simulink model "Rebuild"  (R2024b)
settings: Solver=VariableStepAuto  StartTime=0.0  StopTime=12  RelTol=1e-3
values from neighbouring files (symbols this model uses):
  A = 1.1    [RT14e_Parameters.m]    (also in RT15e_Parameters.m = 1.088; RT15evo_Parameters.m = 1.088)
  Aero_balance = 55    [RT14e_Parameters.m]    (also in RT15e_Parameters.m; RT15evo_Parameters.m)
  Aeromaps_ON = 0    [SIM_setup.m]
  air_density = 1.2    [SIM_setup.m]
  Balance_FW = Data_FW_STD(1:end,2)    [RT15e_Parameters.m]    (also in RT15evo_Parameters.m)
  Balance_R_11 = Data_R_11(1:end,2)    [RT15e_Parameters.m]    (also in RT15evo_Parameters.m)
  Br_coef_of_friction_F = 0.33    [RT14e_Parameters.m]    (also in RT15e_Parameters.m; RT15evo_Parameters.m)
  Br_coef_of_friction_R = 0.33    [RT14e_Parameters.m]    (also in RT15e_Parameters.m; RT15evo_Parameters.m)
  Br_pistons_area_F = 3617.26/1e6    (= 0.00361726)    [RT14e_Parameters.m]    (also in RT15e_Parameters.m; RT15evo_Parameters.m)
  Br_pistons_area_R = 2026.83/1e6    (= 0.00202683)    [RT14e_Parameters.m]    (also in RT15e_Parameters.m; RT15evo_Parameters.m)
  CdA = 1.31*A    (= 1.441)    [RT14e_Parameters.m]    (also in RT15e_Parameters.m = 1.700544; RT15evo_Parameters.m = 1.700544)
  CdA_FW = Data_FW_STD(1:end,3)    [RT15e_Parameters.m]    (also in RT15evo_Parameters.m)
  CdA_R_11 = Data_R_11(1:end,3)    [RT15e_Parameters.m]    (also in RT15evo_Parameters.m)
  ClA = 3.3*A    (= 3.63)    [RT14e_Parameters.m]    (also in RT15e_Parameters.m = 4.36288; RT15evo_Parameters.m = 4.36288)
  ClA_FW = Data_FW_STD(1:end,4)    [RT15e_Parameters.m]    (also in RT15evo_Parameters.m)
  ClA_R_11 = Data_R_11(1:end,4)    [RT15e_Parameters.m]    (also in RT15evo_Parameters.m)
  CoG_z = 0.35    [RT14e_Parameters.m]    (also in RT15e_Parameters.m = 0.28495; RT15evo_Parameters.m = 0.28495)
  Default_Fz_FL = Default_Fz_F/2 + (Default_Fz_F*CoG_y/Track_Front)    [RT14e_Parameters.m]    (also in RT15e_Parameters.m; RT15evo_Parameters.m)
  Default_Fz_FR = Default_Fz_F/2 - (Default_Fz_F*CoG_y/Track_Front)    [RT14e_Parameters.m]    (also in RT15e_Parameters.m; RT15evo_Parameters.m)
  Default_Fz_RL = Default_Fz_R/2 + (Default_Fz_R*CoG_y/Track_Rear)    [RT14e_Parameters.m]    (also in RT15e_Parameters.m; RT15evo_Parameters.m)
  Default_Fz_RR = Default_Fz_R/2 - (Default_Fz_R*CoG_y/Track_Rear)    [RT14e_Parameters.m]    (also in RT15e_Parameters.m; RT15evo_Parameters.m)
  Effective_br_disk_r_F = 0.0905    [RT14e_Parameters.m]    (also in RT15e_Parameters.m; RT15evo_Parameters.m)
  Effective_br_disk_r_R = 0.0895    [RT14e_Parameters.m]    (also in RT15e_Parameters.m; RT15evo_Parameters.m)
  Front_brake_balance = 0.0    (= 0)    [RT14e_Parameters.m]    (also in RT15e_Parameters.m; RT15evo_Parameters.m)
  Front_brake_pump_area = 153.94    [RT14e_Parameters.m]    (also in RT15e_Parameters.m; RT15evo_Parameters.m)
  Front_desired_brake_p_balance = 0.6    [RT14e_Parameters.m]    (also in RT15e_Parameters.m; RT15evo_Parameters.m)
  FW_Setup = Data_FW_STD(1:end,1)    [RT15e_Parameters.m]    (also in RT15evo_Parameters.m)
  Fx = Data_Fx(2:end,3:end)    [RT14e_Parameters.m]    (also in RT15e_Parameters.m; RT15evo_Parameters.m)
  Fy = Data_Fy(2:end,3:end)    [RT14e_Parameters.m]    (also in RT15e_Parameters.m; RT15evo_Parameters.m)
  Fz = Data_Fy(2:end,2)    [RT14e_Parameters.m]    (also in RT15e_Parameters.m; RT15evo_Parameters.m)
  g = 9.81    [SIM_setup.m]
  Gear_ratio = 12.9    [RT14e_Parameters.m]    (also in RT15e_Parameters.m; RT15evo_Parameters.m)
  Iz_wehicle = 120    [RT14e_Parameters.m]    (also in RT15e_Parameters.m; RT15evo_Parameters.m)
  Iz_wheel = 0.15    [RT14e_Parameters.m]    (also in RT15e_Parameters.m; RT15evo_Parameters.m)
  Lf = Wheelbase - CoG_x    (= 0.77)    [RT14e_Parameters.m]    (also in RT15e_Parameters.m = 0.7504; RT15evo_Parameters.m = 0.7504)
  LLTD = 0.45    [RT14e_Parameters.m]    (also in RT15e_Parameters.m = 0.55; RT15evo_Parameters.m = 0.55)
  Lock_brake_balance = false    [RT14e_Parameters.m]    (also in RT15e_Parameters.m; RT15evo_Parameters.m)
  Lr = Wheelbase - Lf    (= 0.755)    [RT14e_Parameters.m]    (also in RT15e_Parameters.m = 0.7746; RT15evo_Parameters.m = 0.7746)
  Mass = Vehicle_mass + Driver_mass    (= 290)    [RT14e_Parameters.m]    (also in RT15e_Parameters.m = 265; RT15evo_Parameters.m)
  Motor_maximum_power = 35366    [RT14e_Parameters.m]    (also in RT15e_Parameters.m; RT15evo_Parameters.m)
  RB_torque_setting_1 = -2    [RT14e_Parameters.m]    (also in RT15e_Parameters.m; RT15evo_Parameters.m)
  RB_torque_setting_10 = -20    [RT14e_Parameters.m]    (also in RT15e_Parameters.m; RT15evo_Parameters.m)
  RB_torque_setting_2 = -4    [RT14e_Parameters.m]    (also in RT15e_Parameters.m; RT15evo_Parameters.m)
  RB_torque_setting_3 = -6    [RT14e_Parameters.m]    (also in RT15e_Parameters.m; RT15evo_Parameters.m)
  RB_torque_setting_4 = -8    [RT14e_Parameters.m]    (also in RT15e_Parameters.m; RT15evo_Parameters.m)
  RB_torque_setting_5 = -10    [RT14e_Parameters.m]    (also in RT15e_Parameters.m; RT15evo_Parameters.m)
  RB_torque_setting_6 = -12    [RT14e_Parameters.m]    (also in RT15e_Parameters.m; RT15evo_Parameters.m)
  RB_torque_setting_7 = -14    [RT14e_Parameters.m]    (also in RT15e_Parameters.m; RT15evo_Parameters.m)
  RB_torque_setting_8 = -16    [RT14e_Parameters.m]    (also in RT15e_Parameters.m; RT15evo_Parameters.m)
  RB_torque_setting_9 = -18    [RT14e_Parameters.m]    (also in RT15e_Parameters.m; RT15evo_Parameters.m)
  Rear_brake_pump_area = 198.56    [RT14e_Parameters.m]    (also in RT15e_Parameters.m; RT15evo_Parameters.m)
  Roll_Angle_11 = Data_R_11(1:end,1)    [RT15e_Parameters.m]    (also in RT15evo_Parameters.m)
  SA = Data_Fy(1,3:end)    [RT14e_Parameters.m]    (also in RT15e_Parameters.m; RT15evo_Parameters.m)
  SR = Data_Fx(1,3:end)    [RT14e_Parameters.m]    (also in RT15e_Parameters.m; RT15evo_Parameters.m)
  start_acc_x = double(start_acc_x_ts.Data)    [SIM_setup.m]
  start_acc_y = double(start_acc_y_ts.Data)    [SIM_setup.m]
  start_time = 1188    [SIM_setup.m]
  start_velocity_x = double(start_velocity_x_ts.Data)    [SIM_setup.m]
  start_velocity_y = double(start_velocity_y_ts.Data)    [SIM_setup.m]
  start_yaw_acc = double(start_yaw_acc_ts.Data)    [SIM_setup.m]
  start_yaw_rate = double(start_yaw_rate_ts.Data)    [SIM_setup.m]
  Static_Camber_FL = 0    [RT14e_Parameters.m]    (also in RT15e_Parameters.m; RT15evo_Parameters.m)
  Static_Camber_FR = 0    [RT14e_Parameters.m]    (also in RT15e_Parameters.m; RT15evo_Parameters.m)
  Static_Camber_RL = 0    [RT14e_Parameters.m]    (also in RT15e_Parameters.m; RT15evo_Parameters.m)
  Static_Camber_RR = 0    [RT14e_Parameters.m]    (also in RT15e_Parameters.m; RT15evo_Parameters.m)
  Static_Toe_FL = 0    [RT14e_Parameters.m]    (also in RT15e_Parameters.m; RT15evo_Parameters.m)
  Static_Toe_FR = 0    [RT14e_Parameters.m]    (also in RT15e_Parameters.m; RT15evo_Parameters.m)
  Static_Toe_RL = 0    [RT14e_Parameters.m]    (also in RT15e_Parameters.m; RT15evo_Parameters.m)
  Static_Toe_RR = 0    [RT14e_Parameters.m]    (also in RT15e_Parameters.m; RT15evo_Parameters.m)
  Steering_Angle_FL = Data_Steering(1:end,2)    [RT14e_Parameters.m]    (also in RT15e_Parameters.m; RT15evo_Parameters.m)
  Steering_Angle_FR = Data_Steering(1:end,3)    [RT14e_Parameters.m]    (also in RT15e_Parameters.m; RT15evo_Parameters.m)
  Steering_Wheel_Angle = Data_Steering(1:end,1)    [RT14e_Parameters.m]    (also in RT15e_Parameters.m; RT15evo_Parameters.m)
  Tire_radius = 0.203    [RT14e_Parameters.m]    (also in RT15e_Parameters.m; RT15evo_Parameters.m)
  Torque_limit_2 = Motor_maximum_torque*0.2    (= 5.82)    [RT14e_Parameters.m]    (also in RT15e_Parameters.m; RT15evo_Parameters.m)
  Torque_limit_3 = Motor_maximum_torque*0.3    (= 8.73)    [RT14e_Parameters.m]    (also in RT15e_Parameters.m; RT15evo_Parameters.m)
  Torque_limit_4 = Motor_maximum_torque*0.4    (= 11.64)    [RT14e_Parameters.m]    (also in RT15e_Parameters.m; RT15evo_Parameters.m)
  Torque_limit_5 = Motor_maximum_torque*0.5    (= 14.55)    [RT14e_Parameters.m]    (also in RT15e_Parameters.m; RT15evo_Parameters.m)
  Torque_limit_6 = Motor_maximum_torque*0.6    (= 17.46)    [RT14e_Parameters.m]    (also in RT15e_Parameters.m; RT15evo_Parameters.m)
  Torque_limit_7 = Motor_maximum_torque*0.7    (= 20.37)    [RT14e_Parameters.m]    (also in RT15e_Parameters.m; RT15evo_Parameters.m)
  Torque_limit_8 = Motor_maximum_torque*0.8    (= 23.28)    [RT14e_Parameters.m]    (also in RT15e_Parameters.m; RT15evo_Parameters.m)
  Torque_limit_9 = 29.1    [RT14e_Parameters.m]    (also in RT15e_Parameters.m; RT15evo_Parameters.m)
  Torque_limit_max = Motor_maximum_torque    (= 29.1)    [RT14e_Parameters.m]    (also in RT15e_Parameters.m; RT15evo_Parameters.m)
  Torque_limit_min = Motor_maximum_torque*0.1    (= 2.91)    [RT14e_Parameters.m]    (also in RT15e_Parameters.m; RT15evo_Parameters.m)
  Torque_limit_set = 10    [RT14e_Parameters.m]    (also in RT15e_Parameters.m; RT15evo_Parameters.m)
  Track_Front = 1.2    [RT14e_Parameters.m]    (also in RT15e_Parameters.m; RT15evo_Parameters.m)
  Track_Rear = 1.18    [RT14e_Parameters.m]    (also in RT15e_Parameters.m; RT15evo_Parameters.m)
  TV_ON = 0    [SIM_setup.m]
  TV_RB_understeer_gradient_1 = -0.5    [RT14e_Parameters.m]    (also in RT15e_Parameters.m; RT15evo_Parameters.m)
  TV_RB_understeer_gradient_10 = 0.005    [RT14e_Parameters.m]    (also in RT15e_Parameters.m; RT15evo_Parameters.m)
  TV_RB_understeer_gradient_2 = -0.1    [RT14e_Parameters.m]    (also in RT15e_Parameters.m; RT15evo_Parameters.m)
  TV_RB_understeer_gradient_3 = 0.08    [RT14e_Parameters.m]    (also in RT15e_Parameters.m; RT15evo_Parameters.m)
  TV_RB_understeer_gradient_4 = 0.06    [RT14e_Parameters.m]    (also in RT15e_Parameters.m; RT15evo_Parameters.m)
  TV_RB_understeer_gradient_5 = 0.05    [RT14e_Parameters.m]    (also in RT15e_Parameters.m; RT15evo_Parameters.m)
  TV_RB_understeer_gradient_6 = 0.04    [RT14e_Parameters.m]    (also in RT15e_Parameters.m; RT15evo_Parameters.m)
  TV_RB_understeer_gradient_7 = 0.03    [RT14e_Parameters.m]    (also in RT15e_Parameters.m; RT15evo_Parameters.m)
  TV_RB_understeer_gradient_8 = 0.02    [RT14e_Parameters.m]    (also in RT15e_Parameters.m; RT15evo_Parameters.m)
  TV_RB_understeer_gradient_9 = 0.01    [RT14e_Parameters.m]    (also in RT15e_Parameters.m; RT15evo_Parameters.m)
  TV_understeer_gradient_1 = -0.5    [RT14e_Parameters.m]    (also in RT15e_Parameters.m; RT15evo_Parameters.m)
  TV_understeer_gradient_10 = 0.002    [RT14e_Parameters.m]    (also in RT15e_Parameters.m; RT15evo_Parameters.m)
  TV_understeer_gradient_2 = -0.1    [RT14e_Parameters.m]    (also in RT15e_Parameters.m; RT15evo_Parameters.m)
  TV_understeer_gradient_3 = 0.06    [RT14e_Parameters.m]    (also in RT15e_Parameters.m; RT15evo_Parameters.m)
  TV_understeer_gradient_4 = 0.05    [RT14e_Parameters.m]    (also in RT15e_Parameters.m; RT15evo_Parameters.m)
  TV_understeer_gradient_5 = 0.04    [RT14e_Parameters.m]    (also in RT15e_Parameters.m; RT15evo_Parameters.m)
  TV_understeer_gradient_6 = 0.03    [RT14e_Parameters.m]    (also in RT15e_Parameters.m; RT15evo_Parameters.m)
  TV_understeer_gradient_7 = 0.02    [RT14e_Parameters.m]    (also in RT15e_Parameters.m; RT15evo_Parameters.m)
  TV_understeer_gradient_8 = 0.01    [RT14e_Parameters.m]    (also in RT15e_Parameters.m; RT15evo_Parameters.m)
  TV_understeer_gradient_9 = 0.005    [RT14e_Parameters.m]    (also in RT15e_Parameters.m; RT15evo_Parameters.m)
  Vx_APPS_ON = 1    [SIM_setup.m]
  Wheel_rolling_resistance = 0.055    [RT14e_Parameters.m]    (also in RT15e_Parameters.m; RT15evo_Parameters.m)
  Wheelbase = 1.525    [RT14e_Parameters.m]    (also in RT15e_Parameters.m; RT15evo_Parameters.m)
undefined symbols (not defined in the file or in its folder): Actual_Torque_Value_RL, Actual_Torque_Value_RR, aero_balance, APPS, Brake_Pressure_Front, Brake_Pressure_Rear, Cl, lateral_load_transfer_distribution, maths_GPS_Velocity, Max_Torque, rad, s, Steering_position, tire_radius, wheel_base, Wheel_Speed_RL, Wheel_Speed_RR, Xsens_MTI_670_accX, Xsens_MTI_670_accY, Xsens_MTI_670_gyrZ
libraries: simulink x30, simulink_extras x11, slpidlib x9, dspstat3 x4, slrealtimeloglib x1, aerolibconvert2 x1
(part 5 of 6)

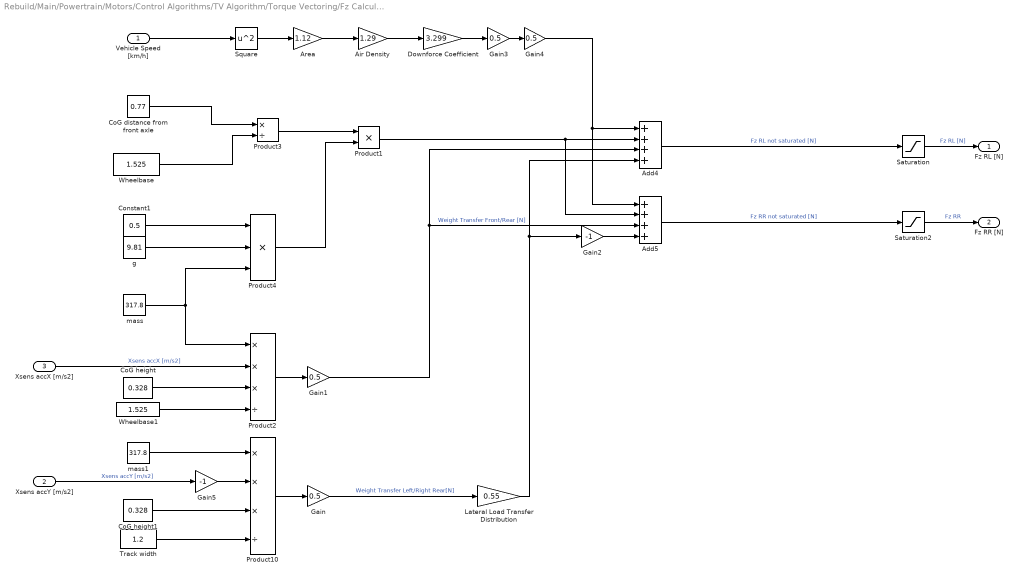
== system Rebuild/Main/Powertrain/Motors/Control Algorithms/TV Algorithm/Torque Vectoring/Fz Calculation ==
  Vehicle Speed [km/h] : Inport
  Xsens accY [m/s2] : Inport  Port=2
  Xsens accX [m/s2] : Inport  Port=3
  Add4 : Sum  Inputs=++++
  Add5 : Sum  Inputs=++++
  Air Density : Gain  Gain=1.29
  Area : Gain  Gain=1.12
  CoG distance from front axle : Constant  Value=0.77
  CoG height : Constant  Value=0.328
  CoG height1 : Constant  Value=0.328
  Constant1 : Constant  Value=0.5
  Downforce Coefficient : Gain  Gain=3.299
  Gain{,1,3..4} (4 alike) : Gain  Gain=0.5
  Gain2 : Gain  Gain=-1
  Gain5 : Gain  Gain=-1
  Lateral Load Transfer Distribution : Gain  Gain=0.55
  Product1 : Product
  Product10 : Product  Inputs=***/
  Product2 : Product  Inputs=***/
  Product3 : Product  Inputs=*/
  Product4 : Product  Inputs=3
  Saturation : Saturate  UpperLimit=10000  LowerLimit=0
  Saturation2 : Saturate  UpperLimit=10000  LowerLimit=0
  Square : Math  Operator=square
  Track width : Constant  Value=1.2
  Wheelbase : Constant  Value=1.525
  Wheelbase1 : Constant  Value=1.525
  g : Constant  Value=9.81
  mass : Constant  Value=317.8
  mass1 : Constant  Value=317.8
  Fz RL [N] : Outport
  Fz RR [N] : Outport  Port=2
  wires:
  Xsens accX [m/s2]/1 -> Product2/2  "Xsens accX [m/s2]"
  Xsens accY [m/s2]/1 -> Gain5/1  "Xsens accY [m/s2]"
  Add5/1 -> Saturation2/1  "Fz RR not saturated [N]"
  Saturation2/1 -> Fz RR [N]/1  "Fz RR"
  Saturation/1 -> Fz RL [N]/1  "Fz RL [N]"
  Add4/1 -> Saturation/1  "Fz RL not saturated [N]"
  Product2/1 -> Gain1/1
  Product3/1 -> Product1/1
  CoG distance from front axle/1 -> Product3/1
  Wheelbase1/1 -> Product2/4
  CoG height/1 -> Product2/3
  mass/1 -> Product4/3, Product2/1
  Product10/1 -> Gain/1
  Constant1/1 -> Product4/1
  Track width/1 -> Product10/4
  g/1 -> Product4/2
  Product4/1 -> Product1/2
  Wheelbase/1 -> Product3/2
  CoG height1/1 -> Product10/3
  mass1/1 -> Product10/1
  Gain/1 -> Lateral Load Transfer Distribution/1  "Weight Transfer Left/Right Rear[N]"
  Gain1/1 -> Add4/3, Add5/3  "Weight Transfer Front/Rear [N]"
  Lateral Load Transfer Distribution/1 -> Add4/4, Gain2/1
  Product1/1 -> Add4/2, Add5/2
  Gain2/1 -> Add5/4
  Vehicle Speed [km/h]/1 -> Square/1
  Square/1 -> Area/1
  Area/1 -> Air Density/1
  Air Density/1 -> Downforce Coefficient/1
  Gain3/1 -> Gain4/1
  Gain4/1 -> Add5/1, Add4/1
  Downforce Coefficient/1 -> Gain3/1
  Gain5/1 -> Product10/2

== system Rebuild/Main/Powertrain/Motors/Control Algorithms/TV Algorithm/Torque Vectoring/RB Torque Difference Calculation ==
  Desired Yaw Rate TV [deg/s] : Inport
  SWS VD Parameter 4 : Inport  Port=2
  " " : Constant  Value=1.2
  "  " : Constant  Value=13
  "   " : Constant  Value=tire_radius
  Abs : Abs  SaturateOnIntegerOverflow=off
  Compare To Constant : simulink/Logic and Bit Operations/Compare To Constant  relop===  const=1  OutDataTypeStr=boolean
  Compare To Constant1 : simulink/Logic and Bit Operations/Compare To Constant  relop===  const=2  OutDataTypeStr=boolean
  Divide3 : Product  Inputs=**
  Divide4 : Product  Inputs=*/
  Divide5 : Product  Inputs=**
  Gain : Gain  Gain=40
  Gain1 : Gain  Gain=0.5
  Gain2 : Gain  Gain=-1
  OR : Logic  Operator=OR  IconShape=distinctive  AllPortsSameDT=off  OutDataTypeStr=boolean
  Saturation : Saturate  UpperLimit=29.1  LowerLimit=0
  Switch : Switch  Criteria=u2 > Threshold  SaturateOnIntegerOverflow=off  InputSameDT=off
  Torque Difference RB [Nm] : Outport
  wires:
  Gain2/1 -> Switch/1
  Switch/1 -> Torque Difference RB [Nm]/1
  Saturation/1 -> Switch/3, Gain2/1  "Torque Difference [Nm]"
  SWS VD Parameter 4/1 -> Compare To Constant/1, Compare To Constant1/1
  Compare To Constant/1 -> OR/1
  Compare To Constant1/1 -> OR/2
  Abs/1 -> Saturation/1
  Gain1/1 -> Abs/1
  Divide4/1 -> Gain1/1
  "   "/1 -> Divide3/1
  " "/1 -> Divide5/2
  Divide5/1 -> Divide4/2
  "  "/1 -> Divide5/1
  Gain/1 -> Divide3/2
  Desired Yaw Rate TV [deg/s]/1 -> Gain/1
  Divide3/1 -> Divide4/1
  OR/1 -> Switch/2

== system Rebuild/Main/Powertrain/Motors/Control Algorithms/TV Algorithm/Torque Vectoring/RB Yaw Rate Calculation ==
  SWS VD Parameter 4 : Inport
  Wheel Angle F [deg] : Inport  Port=2
  Vehicle Speed [km/h] : Inport  Port=3
  " " : Constant  Value=wheel_base
  Add : Sum
  Divide : Product  Inputs=**/
  Divide1 : Product  Inputs=**
  File Log : slrealtimeloglib/File Log  decimation=1  inputProcessing=Elements as channels (sample based)
  Square : Math  Operator=square
  Understeer Gradeint Selection : Subsystem
  Desired Yaw Rate TV RB [deg/s] : Outport
  wires:
  SWS VD Parameter 4/1 -> Understeer Gradeint Selection/1(SWS VD Parameter 4)
  Wheel Angle F [deg]/1 -> Divide/1
  Add/1 -> Divide/3
  Divide1/1 -> Add/2
  Understeer Gradeint Selection/1(Understeer Gradient) -> Divide1/2
  Square/1 -> Divide1/1
  Vehicle Speed [km/h]/1 -> Divide/2, Square/1
  Divide/1 -> Desired Yaw Rate TV RB [deg/s]/1, File Log/1  "Desired Yaw Rate TV [deg/s]"
  " "/1 -> Add/1

== system Rebuild/Main/Powertrain/Motors/Control Algorithms/TV Algorithm/Torque Vectoring/Subsystem ==
  Torque After TV RL [Nm] not saturated : Inport
  SWS VD Parameter 6 : Inport  Port=2
  Torque After TV RR [Nm] not saturated : Inport  Port=3
  Bus Selector : BusSelector  OutputSignals=Torque After TV RL [Nm],Torque After TV RR [Nm]
  Merge : Merge  Inputs=11
  Switch Case : SwitchCase  CaseConditions={1,2,3,4,5,6,7,8,9,10}
  Switch Case Action Subsystem : Subsystem  TreatAsAtomicUnit=on
  Switch Case Action Subsystem1 : Subsystem  TreatAsAtomicUnit=on
  Switch Case Action Subsystem10 : Subsystem  TreatAsAtomicUnit=on
  Switch Case Action Subsystem2 : Subsystem  TreatAsAtomicUnit=on
  Switch Case Action Subsystem3 : Subsystem  TreatAsAtomicUnit=on
  Switch Case Action Subsystem4 : Subsystem  TreatAsAtomicUnit=on
  Switch Case Action Subsystem5 : Subsystem  TreatAsAtomicUnit=on
  Switch Case Action Subsystem6 : Subsystem  TreatAsAtomicUnit=on
  Switch Case Action Subsystem7 : Subsystem  TreatAsAtomicUnit=on
  Switch Case Action Subsystem8 : Subsystem  TreatAsAtomicUnit=on
  Switch Case Action Subsystem9 : Subsystem  TreatAsAtomicUnit=on
  Torque After TV RL [Nm] : Outport
  Torque After TV RR [Nm] : Outport  Port=2
  wires:
  Switch Case Action Subsystem/1(Out1) -> Merge/1
  Switch Case Action Subsystem1/1(Out1) -> Merge/2
  Switch Case Action Subsystem2/1(Out1) -> Merge/3
  Switch Case Action Subsystem3/1(Out1) -> Merge/4
  Switch Case Action Subsystem4/1(Out1) -> Merge/5
  Switch Case Action Subsystem5/1(Out1) -> Merge/6
  Switch Case Action Subsystem6/1(Out1) -> Merge/7
  Switch Case Action Subsystem7/1(Out1) -> Merge/8
  Switch Case Action Subsystem8/1(Out1) -> Merge/9
  Switch Case Action Subsystem9/1(Out1) -> Merge/10
  Switch Case Action Subsystem10/1(Out1) -> Merge/11
  SWS VD Parameter 6/1 -> Switch Case/1
  Switch Case/1 -> Switch Case Action Subsystem/Action
  Switch Case/2 -> Switch Case Action Subsystem1/Action
  Switch Case/3 -> Switch Case Action Subsystem2/Action
  Switch Case/4 -> Switch Case Action Subsystem3/Action
  Switch Case/5 -> Switch Case Action Subsystem4/Action
  Switch Case/6 -> Switch Case Action Subsystem5/Action
  Switch Case/7 -> Switch Case Action Subsystem6/Action
  Switch Case/8 -> Switch Case Action Subsystem7/Action
  Switch Case/9 -> Switch Case Action Subsystem8/Action
  Switch Case/10 -> Switch Case Action Subsystem9/Action
  Switch Case/11 -> Switch Case Action Subsystem10/Action
  Torque After TV RL [Nm] not saturated/1 -> Switch Case Action Subsystem10/1(Torque After TV RL [Nm] not saturated), Switch Case Action Subsystem9/1(Torque After TV RL [Nm] not saturated), Switch Case Action Subsystem8/1(Torque After TV RL [Nm] not saturated), Switch Case Action Subsystem7/1(Torque After TV RL [Nm] not saturated), Switch Case Action Subsystem6/1(Torque After TV RL [Nm] not saturated), Switch Case Action Subsystem5/1(Torque After TV RL [Nm] not saturated), Switch Case Action Subsystem3/1(Torque After TV RL [Nm] not saturated), Switch Case Action Subsystem1/1(Torque After TV RL [Nm] not saturated), Switch Case Action Subsystem/1(Torque After TV RL [Nm] not saturated), Switch Case Action Subsystem2/1(Torque After TV RL [Nm] not saturated), Switch Case Action Subsystem4/1(Torque After TV RL [Nm] not saturated)
  Torque After TV RR [Nm] not saturated/1 -> Switch Case Action Subsystem/2(Torque After TV RR [Nm] not saturated), Switch Case Action Subsystem1/2(Torque After TV RR [Nm] not saturated), Switch Case Action Subsystem2/2(Torque After TV RR [Nm] not saturated), Switch Case Action Subsystem3/2(Torque After TV RR [Nm] not saturated), Switch Case Action Subsystem4/2(Torque After TV RR [Nm] not saturated), Switch Case Action Subsystem5/2(Torque After TV RR [Nm] not saturated), Switch Case Action Subsystem6/2(Torque After TV RR [Nm] not saturated), Switch Case Action Subsystem7/2(Torque After TV RR [Nm] not saturated), Switch Case Action Subsystem8/2(Torque After TV RR [Nm] not saturated), Switch Case Action Subsystem9/2(Torque After TV RR [Nm] not saturated), Switch Case Action Subsystem10/2(Torque After TV RR [Nm] not saturated)
  Merge/1 -> Bus Selector/1
  Bus Selector/1 -> Torque After TV RL [Nm]/1  "<Torque After TV RL [Nm]>"
  Bus Selector/2 -> Torque After TV RR [Nm]/1  "<Torque After TV RR [Nm]>"

== system Rebuild/Main/Powertrain/Motors/Control Algorithms/TV Algorithm/Torque Vectoring/Subsystem1 ==
  Torque After TV RL [Nm] not saturated : Inport
  Torque After TV RR [Nm] not saturated : Inport  Port=2
  SWS VD Parameter 6 : Inport  Port=3
  Bus Selector : BusSelector  OutputSignals=Torque After TV RL [Nm],Torque After TV RR [Nm]
  Merge : Merge  Inputs=11
  Switch Case : SwitchCase  CaseConditions={1,2,3,4,5,6,7,8,9,10}
  Switch Case Action Subsystem : Subsystem  TreatAsAtomicUnit=on
  Switch Case Action Subsystem1 : Subsystem  TreatAsAtomicUnit=on
  Switch Case Action Subsystem10 : Subsystem  TreatAsAtomicUnit=on
  Switch Case Action Subsystem2 : Subsystem  TreatAsAtomicUnit=on
  Switch Case Action Subsystem3 : Subsystem  TreatAsAtomicUnit=on
  Switch Case Action Subsystem4 : Subsystem  TreatAsAtomicUnit=on
  Switch Case Action Subsystem5 : Subsystem  TreatAsAtomicUnit=on
  Switch Case Action Subsystem6 : Subsystem  TreatAsAtomicUnit=on
  Switch Case Action Subsystem7 : Subsystem  TreatAsAtomicUnit=on
  Switch Case Action Subsystem8 : Subsystem  TreatAsAtomicUnit=on
  Switch Case Action Subsystem9 : Subsystem  TreatAsAtomicUnit=on
  Torque After TV RL [Nm] : Outport
  Torque After TV RR [Nm] : Outport  Port=2
  wires:
  Bus Selector/2 -> Torque After TV RR [Nm]/1  "<Torque After TV RR [Nm]>"
  Bus Selector/1 -> Torque After TV RL [Nm]/1  "<Torque After TV RL [Nm]>"
  Merge/1 -> Bus Selector/1
  Torque After TV RR [Nm] not saturated/1 -> Switch Case Action Subsystem10/2(Torque After TV RR [Nm] not saturated), Switch Case Action Subsystem9/2(Torque After TV RR [Nm] not saturated), Switch Case Action Subsystem8/2(Torque After TV RR [Nm] not saturated), Switch Case Action Subsystem7/2(Torque After TV RR [Nm] not saturated), Switch Case Action Subsystem6/2(Torque After TV RR [Nm] not saturated), Switch Case Action Subsystem5/2(Torque After TV RR [Nm] not saturated), Switch Case Action Subsystem4/2(Torque After TV RR [Nm] not saturated), Switch Case Action Subsystem3/2(Torque After TV RR [Nm] not saturated), Switch Case Action Subsystem2/2(Torque After TV RR [Nm] not saturated), Switch Case Action Subsystem1/2(Torque After TV RR [Nm] not saturated), Switch Case Action Subsystem/2(Torque After TV RR [Nm] not saturated)
  Torque After TV RL [Nm] not saturated/1 -> Switch Case Action Subsystem4/1(Torque After TV RL [Nm] not saturated), Switch Case Action Subsystem2/1(Torque After TV RL [Nm] not saturated), Switch Case Action Subsystem/1(Torque After TV RL [Nm] not saturated), Switch Case Action Subsystem1/1(Torque After TV RL [Nm] not saturated), Switch Case Action Subsystem3/1(Torque After TV RL [Nm] not saturated), Switch Case Action Subsystem5/1(Torque After TV RL [Nm] not saturated), Switch Case Action Subsystem6/1(Torque After TV RL [Nm] not saturated), Switch Case Action Subsystem7/1(Torque After TV RL [Nm] not saturated), Switch Case Action Subsystem8/1(Torque After TV RL [Nm] not saturated), Switch Case Action Subsystem9/1(Torque After TV RL [Nm] not saturated), Switch Case Action Subsystem10/1(Torque After TV RL [Nm] not saturated)
  Switch Case/11 -> Switch Case Action Subsystem10/Action
  Switch Case/10 -> Switch Case Action Subsystem9/Action
  Switch Case/9 -> Switch Case Action Subsystem8/Action
  Switch Case/8 -> Switch Case Action Subsystem7/Action
  Switch Case/7 -> Switch Case Action Subsystem6/Action
  Switch Case/6 -> Switch Case Action Subsystem5/Action
  Switch Case/5 -> Switch Case Action Subsystem4/Action
  Switch Case/4 -> Switch Case Action Subsystem3/Action
  Switch Case/3 -> Switch Case Action Subsystem2/Action
  Switch Case/2 -> Switch Case Action Subsystem1/Action
  Switch Case/1 -> Switch Case Action Subsystem/Action
  SWS VD Parameter 6/1 -> Switch Case/1
  Switch Case Action Subsystem10/1(Out1) -> Merge/11
  Switch Case Action Subsystem9/1(Out1) -> Merge/10
  Switch Case Action Subsystem8/1(Out1) -> Merge/9
  Switch Case Action Subsystem7/1(Out1) -> Merge/8
  Switch Case Action Subsystem6/1(Out1) -> Merge/7
  Switch Case Action Subsystem5/1(Out1) -> Merge/6
  Switch Case Action Subsystem4/1(Out1) -> Merge/5
  Switch Case Action Subsystem3/1(Out1) -> Merge/4
  Switch Case Action Subsystem2/1(Out1) -> Merge/3
  Switch Case Action Subsystem1/1(Out1) -> Merge/2
  Switch Case Action Subsystem/1(Out1) -> Merge/1

== system Rebuild/Main/Powertrain/Motors/Control Algorithms/TV Algorithm/Torque Vectoring/Subsystem2 ==
  Brakes : Inport
  In3 : Inport  Port=2
  AND2 : Logic  IconShape=distinctive  AllPortsSameDT=off  OutDataTypeStr=boolean
  Bus Selector : BusSelector  OutputSignals=Front,Rear
  Compare To Constant3 : simulink/Logic and Bit Operations/Compare To Constant  relop=>=  const=5  OutDataTypeStr=boolean
  Compare To Constant4 : simulink/Logic and Bit Operations/Compare To Constant  relop=>=  const=5  OutDataTypeStr=boolean
  OR : Logic  Operator=OR  IconShape=distinctive  AllPortsSameDT=off  OutDataTypeStr=boolean
  Regen Braking Check : Outport
  wires:
  AND2/1 -> Regen Braking Check/1  "Regen Braking Check"
  Compare To Constant3/1 -> OR/2
  OR/1 -> AND2/1
  Compare To Constant4/1 -> OR/1
  In3/1 -> AND2/2
  Bus Selector/1 -> Compare To Constant4/1  "<Front>"
  Brakes/1 -> Bus Selector/1
  Bus Selector/2 -> Compare To Constant3/1  "<Rear>"

== system Rebuild/Main/Powertrain/Motors/Control Algorithms/TV Algorithm/Torque Vectoring/TV Activation ==
  Wheel Angle F [deg] : Inport
  Vehicle Speed [km/h] : Inport  Port=2
  SWS VD Setup 3 : Inport  Port=3
  Regen Braking Check : Inport  Port=4
  R2D Status : Inport  Port=5
  AND : Logic  Inputs=5  IconShape=distinctive  AllPortsSameDT=off  OutDataTypeStr=boolean
  Compare To Constant : simulink/Logic and Bit Operations/Compare To Constant  relop=>=  const=3  OutDataTypeStr=boolean
  Compare To Constant1 : simulink/Logic and Bit Operations/Compare To Constant  relop=<=  const=-3  OutDataTypeStr=boolean
  Compare To Constant2 : simulink/Logic and Bit Operations/Compare To Constant  relop=>  const=-1  OutDataTypeStr=boolean
  NOT : Logic  Operator=NOT  IconShape=distinctive  AllPortsSameDT=off  OutDataTypeStr=boolean
  OR1 : Logic  Operator=OR  IconShape=distinctive  AllPortsSameDT=off  OutDataTypeStr=boolean
  TV Active : Outport
  wires:
  AND/1 -> TV Active/1
  R2D Status/1 -> AND/2
  SWS VD Setup 3/1 -> AND/1
  Compare To Constant1/1 -> OR1/2
  Compare To Constant/1 -> OR1/1
  Wheel Angle F [deg]/1 -> Compare To Constant/1, Compare To Constant1/1
  Vehicle Speed [km/h]/1 -> Compare To Constant2/1
  Compare To Constant2/1 -> AND/3
  OR1/1 -> AND/4
  Regen Braking Check/1 -> NOT/1
  NOT/1 -> AND/5

== system Rebuild/Main/Powertrain/Motors/Control Algorithms/TV Algorithm/Torque Vectoring/TV RB Activation ==
  R2D Status : Inport
  Regen Braking Check : Inport  Port=2
  Vehicle Speed [km/h] : Inport  Port=3
  SWS VD Setup 4 : Inport  Port=4
  Wheel Angle F [deg] : Inport  Port=5
  AND : Logic  Inputs=5  IconShape=distinctive  AllPortsSameDT=off  OutDataTypeStr=boolean
  Compare To Constant : simulink/Logic and Bit Operations/Compare To Constant  relop=>=  const=3  OutDataTypeStr=boolean
  Compare To Constant1 : simulink/Logic and Bit Operations/Compare To Constant  relop=<=  const=-3  OutDataTypeStr=boolean
  Compare To Constant2 : simulink/Logic and Bit Operations/Compare To Constant  relop=>  const=10  OutDataTypeStr=boolean
  OR1 : Logic  Operator=OR  IconShape=distinctive  AllPortsSameDT=off  OutDataTypeStr=boolean
  TV RB Active : Outport
  wires:
  OR1/1 -> AND/4
  Wheel Angle F [deg]/1 -> Compare To Constant1/1, Compare To Constant/1
  Compare To Constant/1 -> OR1/1
  Compare To Constant1/1 -> OR1/2
  SWS VD Setup 4/1 -> AND/1
  R2D Status/1 -> AND/2
  AND/1 -> TV RB Active/1
  Vehicle Speed [km/h]/1 -> Compare To Constant2/1
  Compare To Constant2/1 -> AND/3
  Regen Braking Check/1 -> AND/5

== system Rebuild/Main/Powertrain/Motors/Control Algorithms/TV Algorithm/Torque Vectoring/Torque Difference Calculation ==
  Desired Yaw Rate TV [deg/s] : Inport
  SWS VD Setup 15 : Inport  Port=2
  SWS VD Parameter 3 : Inport  Port=3
  " " : Constant  Value=1.2
  "  " : Constant  Value=13
  "   " : Constant  Value=tire_radius
  AND : Logic  IconShape=distinctive  AllPortsSameDT=off  OutDataTypeStr=boolean
  Abs : Abs  SaturateOnIntegerOverflow=off
  Compare To Constant : simulink/Logic and Bit Operations/Compare To Constant  relop===  const=1  OutDataTypeStr=boolean
  Compare To Constant1 : simulink/Logic and Bit Operations/Compare To Constant  relop===  const=2  OutDataTypeStr=boolean
  Compare To Constant2 : simulink/Logic and Bit Operations/Compare To Constant  relop===  const=0  OutDataTypeStr=boolean
  Divide3 : Product  Inputs=**
  Divide4 : Product  Inputs=*/
  Divide5 : Product  Inputs=**
  Gain : Gain  Gain=40
  Gain1 : Gain  Gain=0.5
  Gain2 : Gain  Gain=-1
  OR : Logic  Operator=OR  IconShape=distinctive  AllPortsSameDT=off  OutDataTypeStr=boolean
  Saturation : Saturate  UpperLimit=Torque_limit_max  LowerLimit=0
  Switch : Switch  Criteria=u2 > Threshold  SaturateOnIntegerOverflow=off  InputSameDT=off
  Torque Difference [Nm] : Outport
  wires:
  Divide3/1 -> Divide4/1
  Desired Yaw Rate TV [deg/s]/1 -> Gain/1
  Gain/1 -> Divide3/2
  "  "/1 -> Divide5/1
  Divide5/1 -> Divide4/2
  " "/1 -> Divide5/2
  "   "/1 -> Divide3/1
  Divide4/1 -> Gain1/1
  Gain1/1 -> Abs/1
  Abs/1 -> Saturation/1
  Compare To Constant1/1 -> OR/2
  Compare To Constant/1 -> OR/1
  SWS VD Parameter 3/1 -> Compare To Constant1/1, Compare To Constant/1
  Saturation/1 -> Gain2/1, Switch/3  "Torque Difference [Nm]"
  Switch/1 -> Torque Difference [Nm]/1
  Gain2/1 -> Switch/1
  OR/1 -> AND/1
  SWS VD Setup 15/1 -> Compare To Constant2/1
  AND/1 -> Switch/2
  Compare To Constant2/1 -> AND/2

== system Rebuild/Main/Powertrain/Motors/Control Algorithms/TV Algorithm/Torque Vectoring/Yaw Rate Calculation ==
  Wheel Angle F [deg] : Inport
  SWS VD Parameter 3 : Inport  Port=2
  SWS VD Setup 15 : Inport  Port=3
  Vehicle Speed [km/h] : Inport  Port=4
  " " : Constant  Value=wheel_base
  Add : Sum
  Divide : Product  Inputs=**/
  Divide1 : Product  Inputs=**
  Square : Math  Operator=square
  Understeer Gradeint Selection : Subsystem
      settings: PortSchema="{\"entries\":[{\"content\":{\"sides\":[{\"content\":{\"connectorIds\":[\"In1\",\"In2\"]},\"type\":\"ConnectorPlacement.EquallySpacedRectSide\",\"uuid\":\"bbee3044-93c1-4f00-ad8f-ae9545aae918\"},{\"content\":{\"connectorIds\":[\"Out1\"],\"side\":\"RIGHT\"},\"type\":\"ConnectorPlacement.EquallySpacedRectSide\",\"uuid\":\"d52ebedb-cc23-4f58-8da8-d3f4b5fce62c\"},{\"content\":{\"connectorIds\":[\"In3\"],\"side\":\"TOP\"},\"type\":\"ConnectorPlacement.EquallySpacedRectSide\",\"uuid\":\"93c9d09d-d680-478a-b9be-fd64b3374c94\"}]},\"type\":\"ConnectorPlacement.EquallySpacedConnector\",\"uuid\":\"e2c6614b-4230-44de-856f-0f9866b3d36c\"}],\"packageUris\":[\"http://schema.mathworks.com/mf0/Connector/R2020b\"],\"version\":\"1.0\"}"
  Desired Yaw Rate TV [deg/s] : Outport
  wires:
  " "/1 -> Add/1
  Divide/1 -> Desired Yaw Rate TV [deg/s]/1  "Desired Yaw Rate TV [deg/s]"
  Square/1 -> Divide1/1
  Understeer Gradeint Selection/1(Understeer Gradient) -> Divide1/2
  Divide1/1 -> Add/2
  Add/1 -> Divide/3
  Wheel Angle F [deg]/1 -> Divide/1
  SWS VD Parameter 3/1 -> Understeer Gradeint Selection/1(SWS VD Parameter 3)
  SWS VD Setup 15/1 -> Understeer Gradeint Selection/2(SWS VD Setup 15)
  Vehicle Speed [km/h]/1 -> Square/1, Understeer Gradeint Selection/3(Vehicle Speed [km/h]), Divide/2

== system Rebuild/Main/Powertrain/Motors/Control Algorithms/TV Algorithm/Subsystem/Fz Calculation/Fz RL Calculation ==
  a_y : Inport
  a_x : Inport  Port=2
  Add1 : Sum
  Add4 : Sum
  CoG distance from front axle : Constant  Value=0.77
  CoG height : Constant  Value=0.328
  CoG height1 : Constant  Value=0.328
  Constant1 : Constant  Value=0.5
  Gain1 : Gain  Gain=0.5
  Gain2 : Gain  Gain=0.5
  Gain8 : Gain  Gain=lateral_load_transfer_distribution
  Product1 : Product
  Product10 : Product  Inputs=***/
  Product2 : Product  Inputs=***/
  Product3 : Product  Inputs=*/
  Product4 : Product  Inputs=3
  Saturation : Saturate  UpperLimit=10000  LowerLimit=0
  Track width : Constant  Value=1.2
  Wheelbase : Constant  Value=1.525
  Wheelbase1 : Constant  Value=1.525
  g : Constant  Value=9.81
  mass : Constant  Value=317.8
  mass1 : Constant  Value=317.8
  Fz RL : Outport
  wires:
  Wheelbase1/1 -> Product2/4
  Product3/1 -> Product1/1
  CoG distance from front axle/1 -> Product3/1
  Add1/1 -> Add4/1
  Product1/1 -> Add1/1
  g/1 -> Product4/2
  Product4/1 -> Product1/2
  Track width/1 -> Product10/4
  a_y/1 -> Product10/2
  Constant1/1 -> Product4/1
  mass1/1 -> Product10/1
  a_x/1 -> Product2/2
  Wheelbase/1 -> Product3/2
  CoG height/1 -> Product2/3
  CoG height1/1 -> Product10/3
  mass/1 -> Product2/1, Product4/3
  Add4/1 -> Saturation/1
  Saturation/1 -> Fz RL/1  "Fz RL"
  Product2/1 -> Gain1/1
  Product10/1 -> Gain2/1
  Gain1/1 -> Add1/2
  Gain2/1 -> Gain8/1
  Gain8/1 -> Add4/2  "Weight Transfer Left/Right Rear[N]"

== system Rebuild/Main/Powertrain/Motors/Control Algorithms/TV Algorithm/Subsystem/Fz Calculation/Fz RR Calculation ==
  a_y : Inport
  a_x : Inport  Port=2
  Add1 : Sum
  Add4 : Sum  Inputs=+-
  CoG distance from front axle : Constant  Value=0.77
  CoG height : Constant  Value=0.328
  CoG height1 : Constant  Value=0.328
  Constant1 : Constant  Value=0.5
  Gain : Gain  Gain=0.5
  Gain1 : Gain  Gain=0.5
  Gain8 : Gain  Gain=lateral_load_transfer_distribution
  Product1 : Product
  Product10 : Product  Inputs=***/
  Product2 : Product  Inputs=***/
  Product3 : Product  Inputs=*/
  Product4 : Product  Inputs=3
  Saturation : Saturate  UpperLimit=10000  LowerLimit=0
  Track width : Constant  Value=1.2
  Wheelbase : Constant  Value=1.525
  Wheelbase1 : Constant  Value=1.525
  g : Constant  Value=9.81
  mass : Constant  Value=317.8
  mass1 : Constant  Value=317.8
  Fz RR : Outport
  wires:
  Product1/1 -> Add1/1
  mass1/1 -> Product10/1
  CoG height1/1 -> Product10/3
  a_y/1 -> Product10/2
  Wheelbase/1 -> Product3/2
  Product4/1 -> Product1/2
  g/1 -> Product4/2
  Track width/1 -> Product10/4
  Constant1/1 -> Product4/1
  mass/1 -> Product2/1, Product4/3
  Add1/1 -> Add4/1
  a_x/1 -> Product2/2
  CoG height/1 -> Product2/3
  Wheelbase1/1 -> Product2/4
  CoG distance from front axle/1 -> Product3/1
  Product3/1 -> Product1/1
  Add4/1 -> Saturation/1
  Saturation/1 -> Fz RR/1  "Fz RR"
  Product10/1 -> Gain/1
  Product2/1 -> Gain1/1
  Gain/1 -> Gain8/1
  Gain1/1 -> Add1/2
  Gain8/1 -> Add4/2  "Weight Transfer Left/Right Rear[N]"

== system Rebuild/Main/Powertrain/Motors/Control Algorithms/TV Algorithm/Torque Vectoring/RB Yaw Rate Calculation/Understeer Gradeint Selection ==
  SWS VD Parameter 4 : Inport
  Merge1 : Merge  Inputs=11
  Switch Case Action Subsystem11 : Subsystem  TreatAsAtomicUnit=on
  Switch Case Action Subsystem12 : Subsystem  TreatAsAtomicUnit=on
  Switch Case Action Subsystem13 : Subsystem  TreatAsAtomicUnit=on
  Switch Case Action Subsystem14 : Subsystem  TreatAsAtomicUnit=on
  Switch Case Action Subsystem15 : Subsystem  TreatAsAtomicUnit=on
  Switch Case Action Subsystem16 : Subsystem  TreatAsAtomicUnit=on
  Switch Case Action Subsystem17 : Subsystem  TreatAsAtomicUnit=on
  Switch Case Action Subsystem18 : Subsystem  TreatAsAtomicUnit=on
  Switch Case Action Subsystem19 : Subsystem  TreatAsAtomicUnit=on
  Switch Case Action Subsystem20 : Subsystem  TreatAsAtomicUnit=on
  Switch Case Action Subsystem21 : Subsystem  TreatAsAtomicUnit=on
  Switch Case1 : SwitchCase  CaseConditions={1,2,3,4,5,6,7,8,9,10}
  Understeer Gradient : Outport
  wires:
  Merge1/1 -> Understeer Gradient/1
  Switch Case Action Subsystem12/1(Out2) -> Merge1/2
  Switch Case Action Subsystem17/1(Out2) -> Merge1/6
  Switch Case1/7 -> Switch Case Action Subsystem18/Action
  Switch Case Action Subsystem14/1(Out1) -> Merge1/3
  Switch Case1/1 -> Switch Case Action Subsystem11/Action
  Switch Case Action Subsystem11/1(Out1) -> Merge1/1
  Switch Case1/6 -> Switch Case Action Subsystem17/Action
  Switch Case1/4 -> Switch Case Action Subsystem15/Action
  Switch Case1/3 -> Switch Case Action Subsystem14/Action
  Switch Case1/5 -> Switch Case Action Subsystem16/Action
  Switch Case Action Subsystem13/1(Out2) -> Merge1/11
  Switch Case Action Subsystem15/1(Out2) -> Merge1/4
  Switch Case Action Subsystem19/1(Out2) -> Merge1/8
  Switch Case Action Subsystem18/1(Out1) -> Merge1/7
  Switch Case1/8 -> Switch Case Action Subsystem19/Action
  Switch Case Action Subsystem21/1(Out1) -> Merge1/10
  Switch Case Action Subsystem16/1(Out1) -> Merge1/5
  Switch Case Action Subsystem20/1(Out2) -> Merge1/9
  Switch Case1/2 -> Switch Case Action Subsystem12/Action
  Switch Case1/10 -> Switch Case Action Subsystem21/Action
  Switch Case1/9 -> Switch Case Action Subsystem20/Action
  Switch Case1/11 -> Switch Case Action Subsystem13/Action
  SWS VD Parameter 4/1 -> Switch Case1/1

== system Rebuild/Main/Powertrain/Motors/Control Algorithms/TV Algorithm/Torque Vectoring/Subsystem/Switch Case Action Subsystem ==
  Torque After TV RL [Nm] not saturated : Inport
  Torque After TV RR [Nm] not saturated : Inport  Port=2
  Action Port : ActionPort
  Bus Creator : BusCreator  Inputs=2
  Saturation : Saturate  UpperLimit=Torque_limit_min  LowerLimit=0
  Saturation1 : Saturate  UpperLimit=Torque_limit_min  LowerLimit=0
  Out1 : Outport
  wires:
  Torque After TV RL [Nm] not saturated/1 -> Saturation/1
  Torque After TV RR [Nm] not saturated/1 -> Saturation1/1
  Saturation/1 -> Bus Creator/1  "Torque After TV RL [Nm]"
  Saturation1/1 -> Bus Creator/2  "Torque After TV RR [Nm]"
  Bus Creator/1 -> Out1/1

== system Rebuild/Main/Powertrain/Motors/Control Algorithms/TV Algorithm/Torque Vectoring/Subsystem/Switch Case Action Subsystem1 ==
  Torque After TV RL [Nm] not saturated : Inport
  Torque After TV RR [Nm] not saturated : Inport  Port=2
  Action Port : ActionPort
  Bus Creator : BusCreator  Inputs=2
  Saturation : Saturate  UpperLimit=Torque_limit_2  LowerLimit=0
  Saturation1 : Saturate  UpperLimit=Torque_limit_2  LowerLimit=0
  Out1 : Outport
  wires:
  Saturation1/1 -> Bus Creator/2  "Torque After TV RR [Nm]"
  Torque After TV RR [Nm] not saturated/1 -> Saturation1/1
  Saturation/1 -> Bus Creator/1  "Torque After TV RL [Nm]"
  Bus Creator/1 -> Out1/1
  Torque After TV RL [Nm] not saturated/1 -> Saturation/1

== system Rebuild/Main/Powertrain/Motors/Control Algorithms/TV Algorithm/Torque Vectoring/Subsystem/Switch Case Action Subsystem10 ==
  Torque After TV RL [Nm] not saturated : Inport
  Torque After TV RR [Nm] not saturated : Inport  Port=2
  Action Port : ActionPort
  Bus Creator : BusCreator  Inputs=2
  Saturation : Saturate  UpperLimit=Torque_limit_max  LowerLimit=0
  Saturation1 : Saturate  UpperLimit=Torque_limit_max  LowerLimit=0
  Out1 : Outport
  wires:
  Saturation1/1 -> Bus Creator/2  "Torque After TV RR [Nm]"
  Torque After TV RR [Nm] not saturated/1 -> Saturation1/1
  Saturation/1 -> Bus Creator/1  "Torque After TV RL [Nm]"
  Bus Creator/1 -> Out1/1
  Torque After TV RL [Nm] not saturated/1 -> Saturation/1

== system Rebuild/Main/Powertrain/Motors/Control Algorithms/TV Algorithm/Torque Vectoring/Subsystem/Switch Case Action Subsystem2 ==
  Torque After TV RL [Nm] not saturated : Inport
  Torque After TV RR [Nm] not saturated : Inport  Port=2
  Action Port : ActionPort
  Bus Creator : BusCreator  Inputs=2
  Saturation : Saturate  UpperLimit=Torque_limit_3  LowerLimit=0
  Saturation1 : Saturate  UpperLimit=Torque_limit_3  LowerLimit=0
  Out1 : Outport
  wires:
  Saturation1/1 -> Bus Creator/2  "Torque After TV RR [Nm]"
  Torque After TV RR [Nm] not saturated/1 -> Saturation1/1
  Saturation/1 -> Bus Creator/1  "Torque After TV RL [Nm]"
  Bus Creator/1 -> Out1/1
  Torque After TV RL [Nm] not saturated/1 -> Saturation/1

== system Rebuild/Main/Powertrain/Motors/Control Algorithms/TV Algorithm/Torque Vectoring/Subsystem/Switch Case Action Subsystem3 ==
  Torque After TV RL [Nm] not saturated : Inport
  Torque After TV RR [Nm] not saturated : Inport  Port=2
  Action Port : ActionPort
  Bus Creator : BusCreator  Inputs=2
  Saturation : Saturate  UpperLimit=Torque_limit_4  LowerLimit=0
  Saturation1 : Saturate  UpperLimit=Torque_limit_4  LowerLimit=0
  Out1 : Outport
  wires:
  Saturation1/1 -> Bus Creator/2  "Torque After TV RR [Nm]"
  Torque After TV RR [Nm] not saturated/1 -> Saturation1/1
  Saturation/1 -> Bus Creator/1  "Torque After TV RL [Nm]"
  Bus Creator/1 -> Out1/1
  Torque After TV RL [Nm] not saturated/1 -> Saturation/1

== system Rebuild/Main/Powertrain/Motors/Control Algorithms/TV Algorithm/Torque Vectoring/Subsystem/Switch Case Action Subsystem4 ==
  Torque After TV RL [Nm] not saturated : Inport
  Torque After TV RR [Nm] not saturated : Inport  Port=2
  Action Port : ActionPort
  Bus Creator : BusCreator  Inputs=2
  Saturation : Saturate  UpperLimit=Torque_limit_5  LowerLimit=0
  Saturation1 : Saturate  UpperLimit=Torque_limit_5  LowerLimit=0
  Out1 : Outport
  wires:
  Saturation1/1 -> Bus Creator/2  "Torque After TV RR [Nm]"
  Torque After TV RR [Nm] not saturated/1 -> Saturation1/1
  Saturation/1 -> Bus Creator/1  "Torque After TV RL [Nm]"
  Bus Creator/1 -> Out1/1
  Torque After TV RL [Nm] not saturated/1 -> Saturation/1

== system Rebuild/Main/Powertrain/Motors/Control Algorithms/TV Algorithm/Torque Vectoring/Subsystem/Switch Case Action Subsystem5 ==
  Torque After TV RL [Nm] not saturated : Inport
  Torque After TV RR [Nm] not saturated : Inport  Port=2
  Action Port : ActionPort
  Bus Creator : BusCreator  Inputs=2
  Saturation : Saturate  UpperLimit=Torque_limit_6  LowerLimit=0
  Saturation1 : Saturate  UpperLimit=Torque_limit_6  LowerLimit=0
  Out1 : Outport
  wires:
  Saturation1/1 -> Bus Creator/2  "Torque After TV RR [Nm]"
  Torque After TV RR [Nm] not saturated/1 -> Saturation1/1
  Saturation/1 -> Bus Creator/1  "Torque After TV RL [Nm]"
  Bus Creator/1 -> Out1/1
  Torque After TV RL [Nm] not saturated/1 -> Saturation/1

== system Rebuild/Main/Powertrain/Motors/Control Algorithms/TV Algorithm/Torque Vectoring/Subsystem/Switch Case Action Subsystem6 ==
  Torque After TV RL [Nm] not saturated : Inport
  Torque After TV RR [Nm] not saturated : Inport  Port=2
  Action Port : ActionPort
  Bus Creator : BusCreator  Inputs=2
  Saturation : Saturate  UpperLimit=Torque_limit_7  LowerLimit=0
  Saturation1 : Saturate  UpperLimit=Torque_limit_7  LowerLimit=0
  Out1 : Outport
  wires:
  Saturation1/1 -> Bus Creator/2  "Torque After TV RR [Nm]"
  Torque After TV RR [Nm] not saturated/1 -> Saturation1/1
  Saturation/1 -> Bus Creator/1  "Torque After TV RL [Nm]"
  Bus Creator/1 -> Out1/1
  Torque After TV RL [Nm] not saturated/1 -> Saturation/1

== system Rebuild/Main/Powertrain/Motors/Control Algorithms/TV Algorithm/Torque Vectoring/Subsystem/Switch Case Action Subsystem7 ==
  Torque After TV RL [Nm] not saturated : Inport
  Torque After TV RR [Nm] not saturated : Inport  Port=2
  Action Port : ActionPort
  Bus Creator : BusCreator  Inputs=2
  Saturation : Saturate  UpperLimit=Torque_limit_8  LowerLimit=0
  Saturation1 : Saturate  UpperLimit=Torque_limit_8  LowerLimit=0
  Out1 : Outport
  wires:
  Saturation1/1 -> Bus Creator/2  "Torque After TV RR [Nm]"
  Torque After TV RR [Nm] not saturated/1 -> Saturation1/1
  Saturation/1 -> Bus Creator/1  "Torque After TV RL [Nm]"
  Bus Creator/1 -> Out1/1
  Torque After TV RL [Nm] not saturated/1 -> Saturation/1

== system Rebuild/Main/Powertrain/Motors/Control Algorithms/TV Algorithm/Torque Vectoring/Subsystem/Switch Case Action Subsystem8 ==
  Torque After TV RL [Nm] not saturated : Inport
  Torque After TV RR [Nm] not saturated : Inport  Port=2
  Action Port : ActionPort
  Bus Creator : BusCreator  Inputs=2
  Saturation : Saturate  UpperLimit=Torque_limit_9  LowerLimit=0
  Saturation1 : Saturate  UpperLimit=Torque_limit_9  LowerLimit=0
  Out1 : Outport
  wires:
  Saturation1/1 -> Bus Creator/2  "Torque After TV RR [Nm]"
  Torque After TV RR [Nm] not saturated/1 -> Saturation1/1
  Saturation/1 -> Bus Creator/1  "Torque After TV RL [Nm]"
  Bus Creator/1 -> Out1/1
  Torque After TV RL [Nm] not saturated/1 -> Saturation/1

== system Rebuild/Main/Powertrain/Motors/Control Algorithms/TV Algorithm/Torque Vectoring/Subsystem/Switch Case Action Subsystem9 ==
  Torque After TV RL [Nm] not saturated : Inport
  Torque After TV RR [Nm] not saturated : Inport  Port=2
  Action Port : ActionPort
  Bus Creator : BusCreator  Inputs=2
  Saturation : Saturate  UpperLimit=Torque_limit_max  LowerLimit=0
  Saturation1 : Saturate  UpperLimit=Torque_limit_max  LowerLimit=0
  Out1 : Outport
  wires:
  Saturation1/1 -> Bus Creator/2  "Torque After TV RR [Nm]"
  Torque After TV RR [Nm] not saturated/1 -> Saturation1/1
  Saturation/1 -> Bus Creator/1  "Torque After TV RL [Nm]"
  Bus Creator/1 -> Out1/1
  Torque After TV RL [Nm] not saturated/1 -> Saturation/1

== system Rebuild/Main/Powertrain/Motors/Control Algorithms/TV Algorithm/Torque Vectoring/Subsystem1/Switch Case Action Subsystem ==
  Torque After TV RL [Nm] not saturated : Inport
  Torque After TV RR [Nm] not saturated : Inport  Port=2
  Action Port : ActionPort
  Bus Creator : BusCreator  Inputs=2
  Saturation : Saturate  UpperLimit=0  LowerLimit=RB_torque_setting_1
  Saturation1 : Saturate  UpperLimit=0  LowerLimit=RB_torque_setting_1
  Out1 : Outport
  wires:
  Bus Creator/1 -> Out1/1
  Saturation1/1 -> Bus Creator/2  "Torque After TV RR [Nm]"
  Saturation/1 -> Bus Creator/1  "Torque After TV RL [Nm]"
  Torque After TV RR [Nm] not saturated/1 -> Saturation1/1
  Torque After TV RL [Nm] not saturated/1 -> Saturation/1

== system Rebuild/Main/Powertrain/Motors/Control Algorithms/TV Algorithm/Torque Vectoring/Subsystem1/Switch Case Action Subsystem1 ==
  Torque After TV RL [Nm] not saturated : Inport
  Torque After TV RR [Nm] not saturated : Inport  Port=2
  Action Port : ActionPort
  Bus Creator : BusCreator  Inputs=2
  Saturation : Saturate  UpperLimit=0  LowerLimit=RB_torque_setting_2
  Saturation1 : Saturate  UpperLimit=0  LowerLimit=RB_torque_setting_2
  Out1 : Outport
  wires:
  Torque After TV RL [Nm] not saturated/1 -> Saturation/1
  Bus Creator/1 -> Out1/1
  Saturation/1 -> Bus Creator/1  "Torque After TV RL [Nm]"
  Torque After TV RR [Nm] not saturated/1 -> Saturation1/1
  Saturation1/1 -> Bus Creator/2  "Torque After TV RR [Nm]"

== system Rebuild/Main/Powertrain/Motors/Control Algorithms/TV Algorithm/Torque Vectoring/Subsystem1/Switch Case Action Subsystem10 ==
  Torque After TV RL [Nm] not saturated : Inport
  Torque After TV RR [Nm] not saturated : Inport  Port=2
  Action Port : ActionPort
  Bus Creator : BusCreator  Inputs=2
  Saturation : Saturate  UpperLimit=Torque_limit_max  LowerLimit=0
  Saturation1 : Saturate  UpperLimit=Torque_limit_max  LowerLimit=0
  Out1 : Outport
  wires:
  Torque After TV RL [Nm] not saturated/1 -> Saturation/1
  Bus Creator/1 -> Out1/1
  Saturation/1 -> Bus Creator/1  "Torque After TV RL [Nm]"
  Torque After TV RR [Nm] not saturated/1 -> Saturation1/1
  Saturation1/1 -> Bus Creator/2  "Torque After TV RR [Nm]"

== system Rebuild/Main/Powertrain/Motors/Control Algorithms/TV Algorithm/Torque Vectoring/Subsystem1/Switch Case Action Subsystem2 ==
  Torque After TV RL [Nm] not saturated : Inport
  Torque After TV RR [Nm] not saturated : Inport  Port=2
  Action Port : ActionPort
  Bus Creator : BusCreator  Inputs=2
  Saturation : Saturate  UpperLimit=0  LowerLimit=RB_torque_setting_3
  Saturation1 : Saturate  UpperLimit=0  LowerLimit=RB_torque_setting_3
  Out1 : Outport
  wires:
  Torque After TV RL [Nm] not saturated/1 -> Saturation/1
  Bus Creator/1 -> Out1/1
  Saturation/1 -> Bus Creator/1  "Torque After TV RL [Nm]"
  Torque After TV RR [Nm] not saturated/1 -> Saturation1/1
  Saturation1/1 -> Bus Creator/2  "Torque After TV RR [Nm]"
